simulink model "VisionModel_test"  (Simulink 7.6)
settings: Solver=FixedStepDiscrete  StartTime=0.0  StopTime=0  RelTol=1e-3
settings Model: Creator=Administrator  LastModifiedBy=auvt

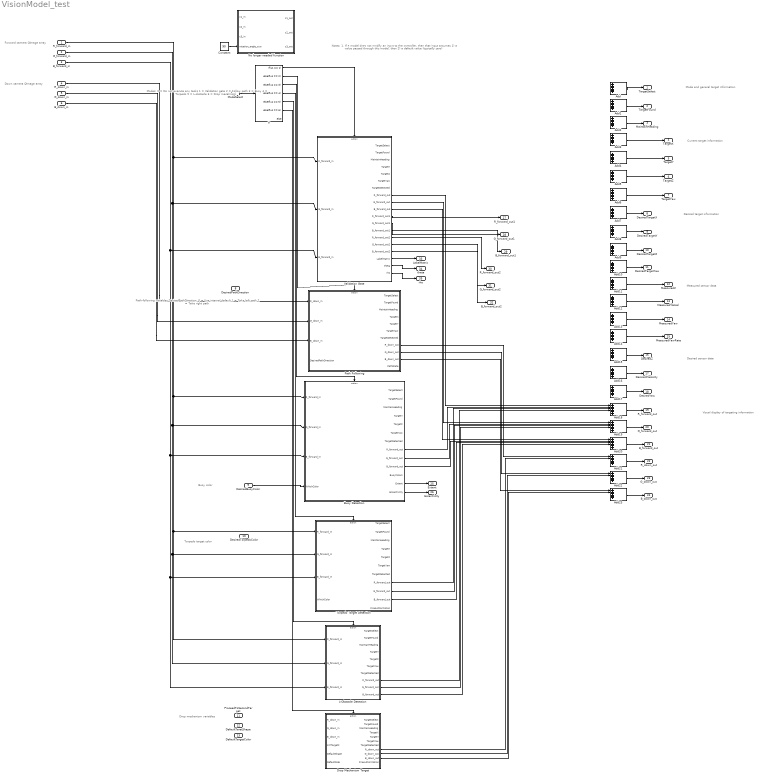
== system VisionModel_test ==
  note: Current target information
  note: Desired target information
  note: Measured sensor data
  note: Mode and general target information
  note: Desired sensor data
  note: Forward camera QImage array
  note: Modes:
      | 0 = Do not execute any tasks
      | 1 = Validation gate
      | 2 = Follow path
      | 3 = Buoy
      | 4 = Torpedo
      | 5 = L-obstacle
      | 6 = Drop mecahnism
  note: Path-following variables
      | DesiredPathDirection:
      | 0 = Use internal default
      | 1 = Take left path
      | 2 = Take right path
  note: Buoy color
  note: Torpedo target color
  note: Drop mechanism variables
  note: Down camera QImage array
  note: Visual display of targeting information
  note: Notes:
      | 1. If a model does not modify an input to the controller,
      | then that input assumes 1) a value passed through this
      | model, then 2) a default value (typically zero)
  R_forward_in : Inport  PortDimensions=[120 160]
  G_forward_in : Inport  Port=2  PortDimensions=[120 160]
  B_forward_in : Inport  Port=3  PortDimensions=[120 160]
  R_down_in : Inport  Port=4  PortDimensions=[120 160]
  G_down_in : Inport  Port=5  PortDimensions=[120 160]
  B_down_in : Inport  Port=6  PortDimensions=[120 160]
  ModeSelect : Inport  Port=7
  DesiredPathDirection : Inport  Port=8
  DesiredBuoyColor : Inport  Port=9
  DesiredTorpedoColor : Inport  Port=10
  ProceedToSecondTarget : Inport  Port=11
  DefaultTaretShape : Inport  Port=12
  DefaultTargetColor : Inport  Port=13
  Add{,1..23} (24 alike) : Sum  Inputs=++++++
  Buoy Detection : Subsystem  TreatAsAtomicUnit=on
  Constant : Constant  Value=90  SampleTime=-1
  Drop Mechanism Target : Subsystem  TreatAsAtomicUnit=on
  If : If  IfExpression=u1 == 1  ElseIfExpressions=u1 == 2, u1 == 3, u1 == 4, u1 == 5, u1 == 6
  L-Obstacle Detection : Subsystem  TreatAsAtomicUnit=on
  No longer needed function : Stateflow chart  TreatAsAtomicUnit=on
  Path Following : Subsystem  TreatAsAtomicUnit=on
  Torpedo Target Detection : Subsystem  TreatAsAtomicUnit=on
  Validation Gate : Subsystem  TreatAsAtomicUnit=on
  TargetSelect : Outport  OutDataTypeStr=double
  TargetFound : Outport  Port=2  OutDataTypeStr=double
  MaintainHeading : Outport  Port=3  OutDataTypeStr=double
  TargetX : Outport  Port=4  OutDataTypeStr=double
  TargetY : Outport  Port=5  OutDataTypeStr=double
  TargetZ : Outport  Port=6  OutDataTypeStr=double
  TargetYaw : Outport  Port=7  OutDataTypeStr=double
  DesiredTargetX : Outport  Port=8  OutDataTypeStr=double
  DesiredTargetY : Outport  Port=9  OutDataTypeStr=double
  DesiredTargetZ : Outport  Port=10  OutDataTypeStr=double
  DesiredTargetYaw : Outport  Port=11  OutDataTypeStr=double
  MeasuredZ : Outport  Port=12  OutDataTypeStr=double
  MeasuredYAccel : Outport  Port=13  OutDataTypeStr=double
  MeasuredYaw : Outport  Port=14  OutDataTypeStr=double
  MeasuredYawRate : Outport  Port=15  OutDataTypeStr=double
  DesiredZ : Outport  Port=16  OutDataTypeStr=double
  DesiredXVelocity : Outport  Port=17  OutDataTypeStr=double
  DesiredYaw : Outport  Port=18  OutDataTypeStr=double
  R_forward_out : Outport  Port=19  OutDataTypeStr=double
  G_forward_out : Outport  Port=20  OutDataTypeStr=double
  B_forward_out : Outport  Port=21  OutDataTypeStr=double
  R_down_out : Outport  Port=22  OutDataTypeStr=double
  G_down_out : Outport  Port=23  OutDataTypeStr=double
  B_down_out : Outport  Port=24  OutDataTypeStr=double
  Extent : Outport  Port=25  OutDataTypeStr=double
  Eccentricity : Outport  Port=26  OutDataTypeStr=double
  R_forward_out1 : Outport  Port=27  OutDataTypeStr=double
  G_forward_out1 : Outport  Port=28  OutDataTypeStr=double
  B_forward_out1 : Outport  Port=29  OutDataTypeStr=double
  R_forward_out2 : Outport  Port=30  OutDataTypeStr=double
  G_forward_out2 : Outport  Port=31  OutDataTypeStr=double
  B_forward_out2 : Outport  Port=32  OutDataTypeStr=double
  LabelMatrix : Outport  Port=33  OutDataTypeStr=double
  theta : Outport  Port=34  OutDataTypeStr=double
  rho : Outport  Port=35  OutDataTypeStr=double
  wires:
  ModeSelect/1 -> If/1
  If/2 -> Path Following/Action
  If/3 -> Buoy Detection/Action
  If/1 -> Validation Gate/Action
  If/4 -> Torpedo Target Detection/Action
  If/5 -> L-Obstacle Detection/Action
  If/6 -> Drop Mechanism Target/Action
  DesiredBuoyColor/1 -> Buoy Detection/4(WhichColor)
  R_down_in/1 -> Path Following/1(R_down_in)
  G_down_in/1 -> Path Following/2(G_down_in)
  B_down_in/1 -> Path Following/3(B_down_in)
  Validation Gate/8(R_forward_out) -> Add18/1
  Add/1 -> TargetSelect/1
  Add1/1 -> TargetFound/1
  Add2/1 -> MaintainHeading/1
  Add3/1 -> TargetX/1
  Add4/1 -> TargetY/1
  Add5/1 -> TargetZ/1
  Add6/1 -> TargetYaw/1
  Add7/1 -> DesiredTargetX/1
  Add8/1 -> DesiredTargetY/1
  Add9/1 -> DesiredTargetZ/1
  Add10/1 -> DesiredTargetYaw/1
  Add11/1 -> MeasuredZ/1
  Add12/1 -> MeasuredYAccel/1
  Add13/1 -> MeasuredYaw/1
  Add14/1 -> MeasuredYawRate/1
  Add15/1 -> DesiredZ/1
  Add16/1 -> DesiredXVelocity/1
  Add17/1 -> DesiredYaw/1
  Add18/1 -> R_forward_out/1
  Add19/1 -> G_forward_out/1
  Add20/1 -> B_forward_out/1
  Add21/1 -> R_down_out/1
  Add22/1 -> G_down_out/1
  Add23/1 -> B_down_out/1
  Buoy Detection/8(R_forward_out) -> Add18/2
  Buoy Detection/9(G_forward_out) -> Add19/2
  Buoy Detection/10(B_forward_out) -> Add20/2
  Torpedo Target Detection/8(R_forward_out) -> Add18/3
  Torpedo Target Detection/9(G_forward_out) -> Add19/3
  Torpedo Target Detection/10(B_forward_out) -> Add20/3
  L-Obstacle Detection/8(R_forward_out) -> Add18/4
  L-Obstacle Detection/9(G_forward_out) -> Add19/4
  L-Obstacle Detection/10(B_forward_out) -> Add20/4
  Constant/1 -> No longer needed function/4(rotation_angle_ccw)
  Path Following/8(R_down_out) -> Add21/1
  Path Following/9(G_down_out) -> Add22/1
  Path Following/10(B_down_out) -> Add23/1
  Drop Mechanism Target/8(R_down_out) -> Add21/2
  Drop Mechanism Target/9(G_down_out) -> Add22/2
  Drop Mechanism Target/10(B_down_out) -> Add23/2
  Validation Gate/9(G_forward_out) -> Add19/1
  Validation Gate/10(B_forward_out) -> Add20/1
  R_forward_in/1 -> Validation Gate/1(R_forward_in), Buoy Detection/1(R_forward_in), Torpedo Target Detection/1(R_forward_in), L-Obstacle Detection/1(R_forward_in)
  G_forward_in/1 -> Validation Gate/2(G_forward_in), Buoy Detection/2(G_forward_in), Torpedo Target Detection/2(G_forward_in), L-Obstacle Detection/2(G_forward_in)
  B_forward_in/1 -> Validation Gate/3(B_forward_in), Buoy Detection/3(B_forward_in), Torpedo Target Detection/3(B_forward_in), L-Obstacle Detection/3(B_forward_in)
  Buoy Detection/12(Extent) -> Extent/1
  Buoy Detection/13(Eccentricity) -> Eccentricity/1
  Validation Gate/11(R_forward_out1) -> R_forward_out1/1
  Validation Gate/12(G_forward_out1) -> G_forward_out1/1
  Validation Gate/13(B_forward_out1) -> B_forward_out1/1
  Validation Gate/14(R_forward_out2) -> R_forward_out2/1
  Validation Gate/15(G_forward_out2) -> G_forward_out2/1
  Validation Gate/16(B_forward_out2) -> B_forward_out2/1
  Validation Gate/17(LabelMatrix) -> LabelMatrix/1
  Validation Gate/18(theta) -> theta/1
  Validation Gate/19(rho) -> rho/1

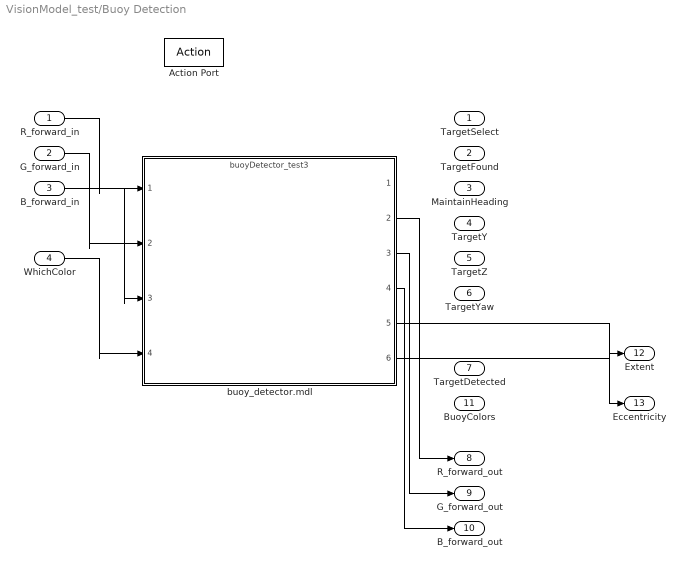
== system VisionModel_test/Buoy Detection ==
  R_forward_in : Inport  PortDimensions=[120 160]
  G_forward_in : Inport  Port=2  PortDimensions=[120 160]
  B_forward_in : Inport  Port=3  PortDimensions=[120 160]
  WhichColor : Inport  Port=4
  Action Port : ActionPort  ActionType=elseif
  buoy_detector.mdl : ModelReference  ModelNameDialog=buoyDetector_test3  SimulationMode=Accelerator  ModelReferenceVersion=1.643  CopyOfModelName=buoyDetector_test3
  TargetSelect : Outport  OutDataTypeStr=double
  TargetFound : Outport  Port=2  OutDataTypeStr=double
  MaintainHeading : Outport  Port=3  OutDataTypeStr=double
  TargetY : Outport  Port=4  OutDataTypeStr=double
  TargetZ : Outport  Port=5  OutDataTypeStr=double
  TargetYaw : Outport  Port=6  OutDataTypeStr=double
  TargetDetected : Outport  Port=7  OutDataTypeStr=double
  R_forward_out : Outport  Port=8  OutDataTypeStr=double  PortDimensions=[120 160]
  G_forward_out : Outport  Port=9  OutDataTypeStr=double  PortDimensions=[120 160]
  B_forward_out : Outport  Port=10  OutDataTypeStr=double  PortDimensions=[120 160]
  BuoyColors : Outport  Port=11  OutDataTypeStr=double
  Extent : Outport  Port=12  OutDataTypeStr=double
  Eccentricity : Outport  Port=13  OutDataTypeStr=double
  wires:
  R_forward_in/1 -> buoy_detector.mdl/1
  G_forward_in/1 -> buoy_detector.mdl/2
  B_forward_in/1 -> buoy_detector.mdl/3
  WhichColor/1 -> buoy_detector.mdl/4
  buoy_detector.mdl/2 -> R_forward_out/1
  buoy_detector.mdl/3 -> G_forward_out/1
  buoy_detector.mdl/4 -> B_forward_out/1
  buoy_detector.mdl/5 -> Eccentricity/1
  buoy_detector.mdl/6 -> Extent/1

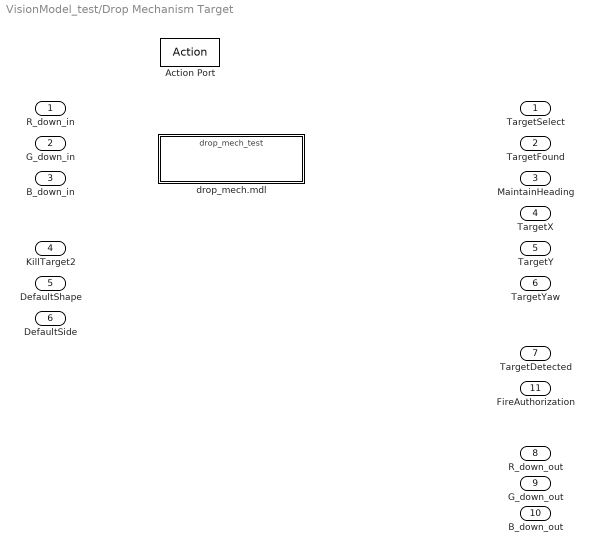
== system VisionModel_test/Drop Mechanism Target ==
  R_down_in : Inport
  G_down_in : Inport  Port=2
  B_down_in : Inport  Port=3
  KillTarget2 : Inport  Port=4
  DefaultShape : Inport  Port=5
  DefaultSide : Inport  Port=6
  Action Port : ActionPort  ActionType=elseif
  drop_mech.mdl : ModelReference  ModelNameDialog=drop_mech_test  SimulationMode=Accelerator  ModelReferenceVersion=1.2  CopyOfModelName=drop_mech_test
  TargetSelect : Outport  OutDataTypeStr=double
  TargetFound : Outport  Port=2  OutDataTypeStr=double
  MaintainHeading : Outport  Port=3  OutDataTypeStr=double
  TargetX : Outport  Port=4  OutDataTypeStr=double
  TargetY : Outport  Port=5  OutDataTypeStr=double
  TargetYaw : Outport  Port=6  OutDataTypeStr=double
  TargetDetected : Outport  Port=7  OutDataTypeStr=double
  R_down_out : Outport  Port=8  OutDataTypeStr=double
  G_down_out : Outport  Port=9  OutDataTypeStr=double
  B_down_out : Outport  Port=10  OutDataTypeStr=double
  FireAuthorization : Outport  Port=11  OutDataTypeStr=double

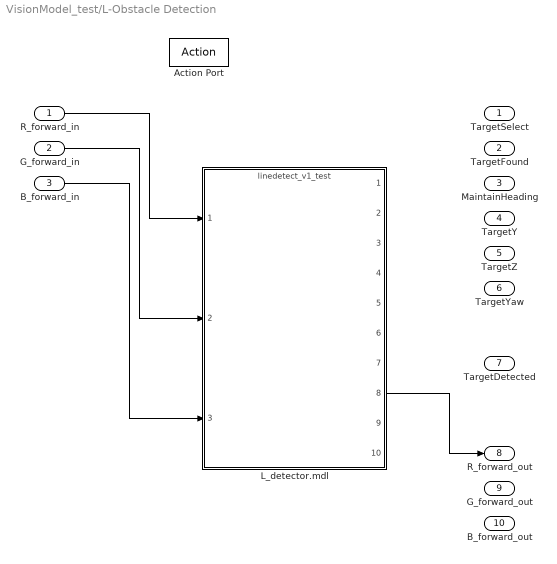
== system VisionModel_test/L-Obstacle Detection ==
  R_forward_in : Inport
  G_forward_in : Inport  Port=2
  B_forward_in : Inport  Port=3
  Action Port : ActionPort  ActionType=elseif
  L_detector.mdl : ModelReference  ModelNameDialog=linedetect_v1_test  SimulationMode=Accelerator  ModelReferenceVersion=1.141  CopyOfModelName=linedetect_v1_test
  TargetSelect : Outport  OutDataTypeStr=double
  TargetFound : Outport  Port=2  OutDataTypeStr=double
  MaintainHeading : Outport  Port=3  OutDataTypeStr=double
  TargetY : Outport  Port=4  OutDataTypeStr=double
  TargetZ : Outport  Port=5  OutDataTypeStr=double
  TargetYaw : Outport  Port=6  OutDataTypeStr=double
  TargetDetected : Outport  Port=7  OutDataTypeStr=double
  R_forward_out : Outport  Port=8  OutDataTypeStr=double
  G_forward_out : Outport  Port=9  OutDataTypeStr=double
  B_forward_out : Outport  Port=10  OutDataTypeStr=double
  wires:
  L_detector.mdl/8 -> R_forward_out/1
  R_forward_in/1 -> L_detector.mdl/1
  G_forward_in/1 -> L_detector.mdl/2
  B_forward_in/1 -> L_detector.mdl/3

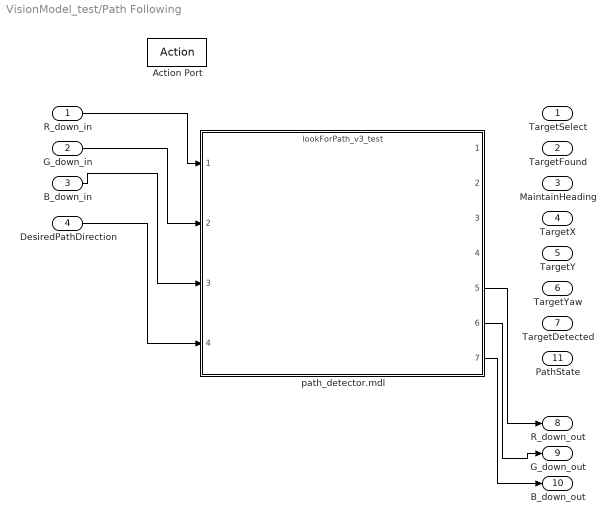
== system VisionModel_test/Path Following ==
  R_down_in : Inport
  G_down_in : Inport  Port=2
  B_down_in : Inport  Port=3
  DesiredPathDirection : Inport  Port=4
  Action Port : ActionPort  ActionType=elseif
  path_detector.mdl : ModelReference  ModelNameDialog=lookForPath_v3_test  SimulationMode=Accelerator  ModelReferenceVersion=1.211  CopyOfModelName=lookForPath_v3_test
  TargetSelect : Outport  OutDataTypeStr=double
  TargetFound : Outport  Port=2  OutDataTypeStr=double
  MaintainHeading : Outport  Port=3  OutDataTypeStr=double
  TargetX : Outport  Port=4  OutDataTypeStr=double
  TargetY : Outport  Port=5  OutDataTypeStr=double
  TargetYaw : Outport  Port=6  OutDataTypeStr=double
  TargetDetected : Outport  Port=7  OutDataTypeStr=double
  R_down_out : Outport  Port=8  OutDataTypeStr=double
  G_down_out : Outport  Port=9  OutDataTypeStr=double
  B_down_out : Outport  Port=10  OutDataTypeStr=double
  PathState : Outport  Port=11  OutDataTypeStr=double
  wires:
  R_down_in/1 -> path_detector.mdl/1
  G_down_in/1 -> path_detector.mdl/2
  B_down_in/1 -> path_detector.mdl/3
  DesiredPathDirection/1 -> path_detector.mdl/4
  path_detector.mdl/5 -> R_down_out/1
  path_detector.mdl/6 -> G_down_out/1
  path_detector.mdl/7 -> B_down_out/1

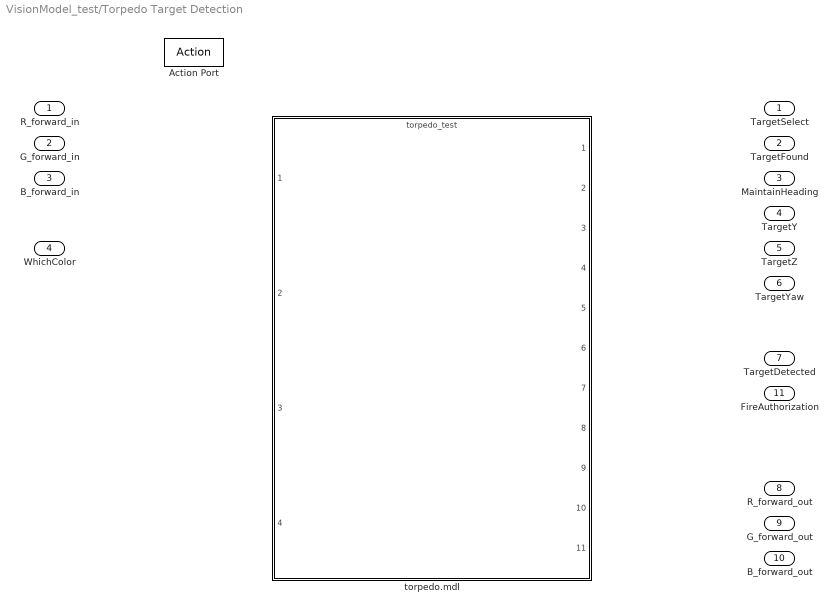
== system VisionModel_test/Torpedo Target Detection ==
  R_forward_in : Inport
  G_forward_in : Inport  Port=2
  B_forward_in : Inport  Port=3
  WhichColor : Inport  Port=4
  Action Port : ActionPort  ActionType=elseif
  torpedo.mdl : ModelReference  ModelNameDialog=torpedo_test  SimulationMode=Accelerator  ModelReferenceVersion=1.58  CopyOfModelName=torpedo_test
  TargetSelect : Outport  OutDataTypeStr=double
  TargetFound : Outport  Port=2  OutDataTypeStr=double
  MaintainHeading : Outport  Port=3  OutDataTypeStr=double
  TargetY : Outport  Port=4  OutDataTypeStr=double
  TargetZ : Outport  Port=5  OutDataTypeStr=double
  TargetYaw : Outport  Port=6  OutDataTypeStr=double
  TargetDetected : Outport  Port=7  OutDataTypeStr=double
  R_forward_out : Outport  Port=8  OutDataTypeStr=double
  G_forward_out : Outport  Port=9  OutDataTypeStr=double
  B_forward_out : Outport  Port=10  OutDataTypeStr=double
  FireAuthorization : Outport  Port=11  OutDataTypeStr=double

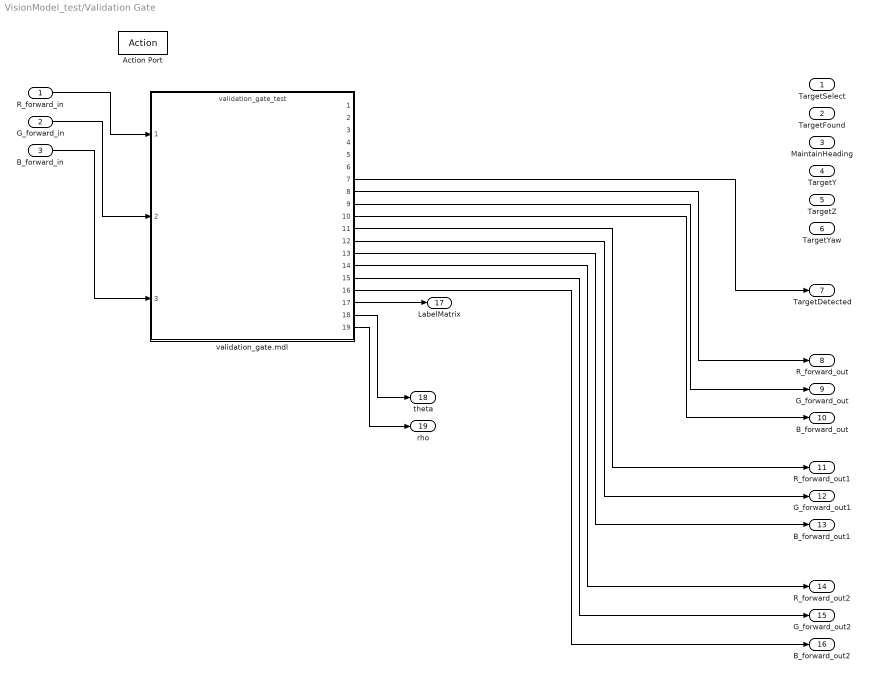
== system VisionModel_test/Validation Gate ==
  R_forward_in : Inport
  G_forward_in : Inport  Port=2
  B_forward_in : Inport  Port=3
  Action Port : ActionPort  ActionType=then
  validation_gate.mdl : ModelReference  ModelNameDialog=validation_gate_test  SimulationMode=Accelerator  ModelReferenceVersion=1.907  CopyOfModelName=validation_gate_test
  TargetSelect : Outport  OutDataTypeStr=double
  TargetFound : Outport  Port=2  OutDataTypeStr=double
  MaintainHeading : Outport  Port=3  OutDataTypeStr=double
  TargetY : Outport  Port=4  OutDataTypeStr=double
  TargetZ : Outport  Port=5  OutDataTypeStr=double
  TargetYaw : Outport  Port=6  OutDataTypeStr=double
  TargetDetected : Outport  Port=7  OutDataTypeStr=double
  R_forward_out : Outport  Port=8  OutDataTypeStr=double
  G_forward_out : Outport  Port=9  OutDataTypeStr=double
  B_forward_out : Outport  Port=10  OutDataTypeStr=double
  R_forward_out1 : Outport  Port=11  OutDataTypeStr=double
  G_forward_out1 : Outport  Port=12  OutDataTypeStr=double
  B_forward_out1 : Outport  Port=13  OutDataTypeStr=double
  R_forward_out2 : Outport  Port=14  OutDataTypeStr=double
  G_forward_out2 : Outport  Port=15  OutDataTypeStr=double
  B_forward_out2 : Outport  Port=16  OutDataTypeStr=double
  LabelMatrix : Outport  Port=17  OutDataTypeStr=double
  theta : Outport  Port=18  OutDataTypeStr=double
  rho : Outport  Port=19  OutDataTypeStr=double
  wires:
  R_forward_in/1 -> validation_gate.mdl/1
  validation_gate.mdl/7 -> TargetDetected/1
  validation_gate.mdl/8 -> R_forward_out/1
  validation_gate.mdl/9 -> G_forward_out/1
  validation_gate.mdl/10 -> B_forward_out/1
  G_forward_in/1 -> validation_gate.mdl/2
  B_forward_in/1 -> validation_gate.mdl/3
  validation_gate.mdl/11 -> R_forward_out1/1
  validation_gate.mdl/12 -> G_forward_out1/1
  validation_gate.mdl/13 -> B_forward_out1/1
  validation_gate.mdl/14 -> R_forward_out2/1
  validation_gate.mdl/15 -> G_forward_out2/1
  validation_gate.mdl/16 -> B_forward_out2/1
  validation_gate.mdl/17 -> LabelMatrix/1
  validation_gate.mdl/18 -> theta/1
  validation_gate.mdl/19 -> rho/1

== matlab function No longer needed function ==
  data: c1_in input double; c2_in input double; c3_in input double; c1_out output double; rotation_angle_ccw input double; c2_out output double; c3_out output double
function [c1_out, c2_out, c3_out] = rotateImage(c1_in, c2_in, c3_in, rotation_angle_ccw)
%#eml

% This function rotates an image in 90 degree increments
%
% Input
%   c1_in = input image component 1 data
%                   Note: Must be a 2-D (single color component) or 3-D
%                     (RGB or similar) array; first two dimensions
%                     specify image height and width, respectively
%   c2_in = input image component 2 data
%   c3_in = input image component 3 data
%
% Output
%   c1_out = output image component 1 data
%   c1_out = output image component 2 data
%   c1_out = output image component 3 data

% Determine loop indices
[m, n, depth] = size(c1_in);


% Initialize output
c1_out = double(zeros([120 160]));
c2_out = double(zeros([120 160]));
c3_out = double(zeros([120 160]));


% Loop
for i = 1:m
    for j = 1:n
        if(rotation_angle_ccw == 0)
            c1_out(i,j,:) = c1_in(i,j,:);
            c2_out(i,j,:) = c2_in(i,j,:);
            c3_out(i,j,:) = c3_in(i,j,:);
        elseif(rotation_angle_ccw == 90)
            c1_out(n-j+1,i,:) = c1_in(i,j,:);
            c2_out(n-j+1,i,:) = c2_in(i,j,:);
            c3_out(n-j+1,i,:) = c3_in(i,j,:);
%        elseif(rotation_angle_ccw == 180)
%            image_out(m-i+1,n-j+1) = image_in(i,j,:);
%        elseif(rotation_angle_ccw == 270)
%            image_out(j,m-i+1) = image_in(i,j,:);
        end
    end
end


return
